simulink model "AltitudeControllerProject"  (R2026b)
settings: Solver=VariableStepAuto  StopTime=30
model workspace (MAT data in the model file):
  g = 9.81
  m = 1.5
undefined symbols (not defined in the file): Discrete, N, R, Time
libraries: slpidlib x1, ctrlSharedLib x1
settings Model: Creator=bosto  LastModifiedBy=bosto

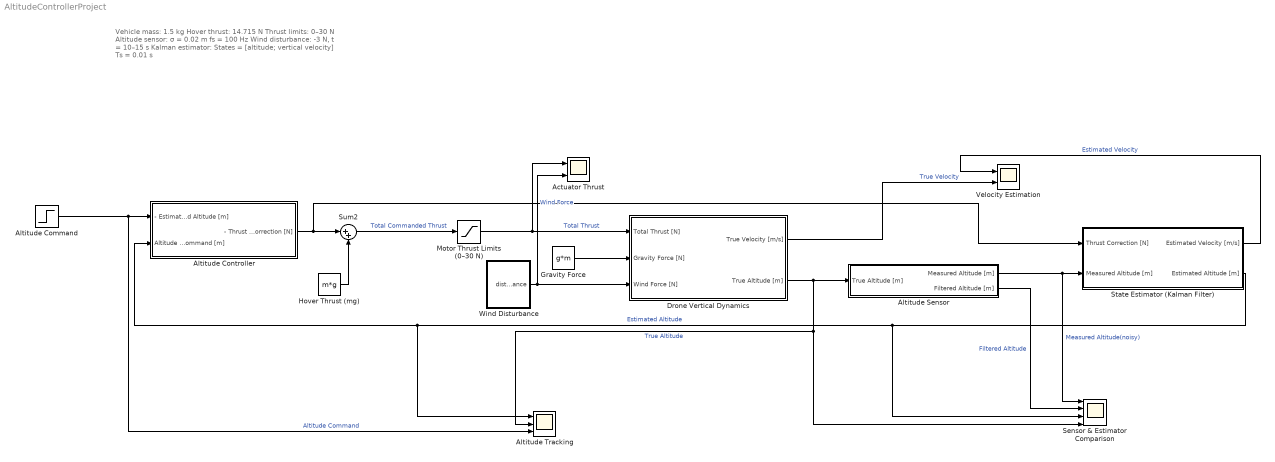
== system AltitudeControllerProject ==
  note: Vehicle mass: 1.5 kg
      | Hover thrust: 14.715 N
      | Thrust limits: 0–30 N
      |
      | Altitude sensor:
      | σ = 0.02 m
      | fs = 100 Hz
      |
      | Wind disturbance:
      | -3 N, t = 10–15 s
      |
      | Kalman estimator:
      | States = [altitude; vertical velocity]
      | Ts = 0.01 s
  Actuator Thrust : Scope  NumInputPorts=2
      settings: ActiveDisplayYMinimum=-7.1717687074829932  ActiveDisplayYMaximum=34.078231292517
  Altitude Command : Step  FinalValue=10  SampleTime=0
  Altitude Controller : Subsystem
  Altitude Sensor : Subsystem
  Altitude Tracking : Scope  NumInputPorts=3
      settings: ActiveDisplayYMinimum=-1.4089981765481037  ActiveDisplayYMaximum=12.477747899037325  DataLoggingVariableName=ScopeData3
  Drone Vertical Dynamics : Subsystem
  "Gravity Force " : Constant  Value=g*m
  Hover Thrust (mg) : Constant  Value=m*g
  Motor Thrust Limits (0–30 N) : Saturate  UpperLimit=30  LowerLimit=0
  Sensor & Estimator Comparison : Scope  NumInputPorts=4
      settings: ActiveDisplayYMinimum=9.9287970603381659  ActiveDisplayYMaximum=10.712908697624938
  State Estimator (Kalman Filter) : Subsystem
  Sum2 : Sum  Inputs=|++
  Velocity Estimation : Scope  NumInputPorts=2
      settings: ActiveDisplayYMinimum=-1.6989208652949748  ActiveDisplayYMaximum=10.973825126247741  DataLoggingVariableName=ScopeData4
  Wind Disturbance : Subsystem
  wires:
  Hover Thrust (mg)/1 -> Sum2/2
  "Gravity Force "/1 -> Drone Vertical Dynamics/2("Gravity Force [N] ")
  Motor Thrust Limits (0–30 N)/1 -> Actuator Thrust/1, Drone Vertical Dynamics/1(Total Thrust [N])  "Total Thrust"
  Sum2/1 -> Motor Thrust Limits (0–30 N)/1  "Total Commanded Thrust"
  Altitude Controller/1(- Thrust Correction [N]) -> Sum2/1, State Estimator (Kalman Filter)/1(Thrust Correction [N])
  Altitude Command/1 -> Altitude Tracking/3, Altitude Controller/1(- Estimated Altitude [m])  "Altitude Command"
  Altitude Sensor/2(Filtered Altitude [m]) -> Sensor & Estimator Comparison/2  "Filtered Altitude"
  Altitude Sensor/1(Measured Altitude [m]) -> Sensor & Estimator Comparison/1, State Estimator (Kalman Filter)/2(Measured Altitude [m])  "Measured Altitude(noisy)"
  State Estimator (Kalman Filter)/1(Estimated Velocity [m/s]) -> Velocity Estimation/1  "Estimated Velocity"
  State Estimator (Kalman Filter)/2(Estimated Altitude [m]) -> Sensor & Estimator Comparison/3, Altitude Tracking/1, Altitude Controller/2(Altitude Command [m])  "Estimated Altitude"
  Wind Disturbance/1(disturbance) -> Drone Vertical Dynamics/3(Wind Force [N]), Actuator Thrust/2  "Wind Force"
  Drone Vertical Dynamics/1(True Velocity [m/s]) -> Velocity Estimation/2  "True Velocity"
  Drone Vertical Dynamics/2(True Altitude [m]) -> Altitude Tracking/2, Sensor & Estimator Comparison/4, Altitude Sensor/1(True Altitude [m])  "True Altitude"

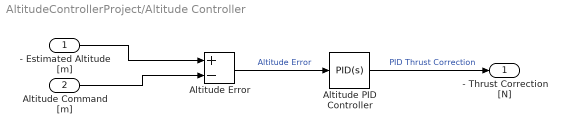
== system AltitudeControllerProject/Altitude Controller ==
  - Estimated Altitude [m] : Inport
  Altitude Command [m] : Inport  Port=2
  Altitude Error : Sum  Inputs=+-
  Altitude PID Controller : slpidlib/PID Controller  Controller=PID  Form=Parallel  TimeDomain=Continuous-time  UseExternalTs=off  SampleTime=-1  IntegratorMethod=Forward Euler  FilterMethod=Forward Euler  ControllerParametersSource=internal  P=34.1948073252816  I=4.38969736985132  UseKiTs=off  D=24.4181996821772  UseExternalDerivativeSource=off  N=10  UseFilter=on  TunerSelectOption=Transfer Function Based (PID Tuner App)  InitialConditionSource=internal  InitialConditionForIntegrator=0  InitialConditionForFilter=0  DifferentiatorICPrevScaledInput=0  ExternalReset=none  TrackingMode=off  Kt=1  LimitOutput=on  SatLimitsSource=internal  UpperSaturationLimit=15.285  LowerSaturationLimit=-14.715  LinearizeAsGain=on  AntiWindupMode=none  Kb=1  LimitIntegrator=off  UpperIntegratorSaturationLimit=inf  LowerIntegratorSaturationLimit=-inf  POutMin=[]  POutMax=[]  IOutMin=[]  IOutMax=[]  DOutMin=[]  DOutMax=[]  NOutMin=[]  NOutMax=[]  SumOutMin=[]  SumOutMax=[]  SaturationOutMin=[]  SaturationOutMax=[]  PParamMin=[]  PParamMax=[]  IParamMin=[]  IParamMax=[]  DParamMin=[]  DParamMax=[]  NParamMin=[]  NParamMax=[]  KbParamMin=[]  KbParamMax=[]  KtParamMin=[]  KtParamMax=[]  KbOutMin=[]  KbOutMax=[]  KtOutMin=[]  KtOutMax=[]  IntegratorOutMin=[]  IntegratorOutMax=[]  FilterOutMin=[]  FilterOutMax=[]  SumI1OutMin=[]  SumI1OutMax=[]  SumI2OutMin=[]  SumI2OutMax=[]  SumI3OutMin=[]  SumI3OutMax=[]  SumI4OutMin=[]  SumI4OutMax=[]  SumDOutMin=[]  SumDOutMax=[]  DifferentiatorOutMin=[]  DifferentiatorOutMax=[]  FilterDiffOutCoefMin=[]  FilterDiffOutCoefMax=[]  ReciprocalOutMin=[]  ReciprocalOutMax=[]  SumDenOutMin=[]  SumDenOutMax=[]  SumNumOutMin=[]  SumNumOutMax=[]  DivideOutMin=[]  DivideOutMax=[]  UdiffTsProdOutMin=[]  UdiffTsProdOutMax=[]  NTsProdOutMin=[]  NTsProdOutMax=[]  UintegralTsProdOutMin=[]  UintegralTsProdOutMax=[]  UngainTsProdOutMin=[]  UngainTsProdOutMax=[]  ClampingZeroOutDataTypeStr=Inherit: Inherit via back propagation  ClampingZeroOutMin=[]  ClampingZeroOutMax=[]  FilterDenConstantOutDataTypeStr=Inherit: Inherit via back propagation  FilterDenConstantOutMin=[]  FilterDenConstantOutMax=[]  PCopyOutDataTypeStr=Inherit: Inherit via back propagation  PCopyOutMin=[]  PCopyOutMax=[]  NCopyOutDataTypeStr=Inherit: Inherit via back propagation  NCopyOutMin=[]  NCopyOutMax=[]  IntegratorContinuousStateAttributes=''  IntegratorStateMustResolveToSignalObject=off  IntegratorRTWStateStorageClass=Auto  FilterContinuousStateAttributes=''  FilterStateMustResolveToSignalObject=off  FilterRTWStateStorageClass=Auto  ParallelPVariant=InternalParameters  IdealPVariant=Disabled  IVariant=InternalParameters  DVariant=InternalParameters  IntegratorVariant=Continuous  SatVariant=Enabled  AWVariant=Passthrough  PCopyVariant=Disabled  TRVariant=Disabled  FdbkBlocksVariant=Forward  IdealPFdbkVariant=Disabled  SatFdbkVariant=Disabled  DerivativeFilterVariant=ContFilter  NVariant=InternalParameters  NCopyVariant=Disabled  FilterICVariant=InternalICsFilter  IntegratorICVariant=InternalICs  ExternalResetVariant=Disabled  TRSumVariant=Passthrough  SumFdbkVariant=Disabled  SumVariant=Sum_PID  TsampFilterVariant=InternalTs  TsampNgainVariant=Passthrough  TsampIntegralVariant=Disabled_SignalSpec  ExternalSaturationOutDataTypeStr=Inherit: Same as second input  DerivativeSourceVariant=ErrorSignal  PreIntVariant=InternalPreInt
  - Thrust Correction [N] : Outport
  wires:
  - Estimated Altitude [m]/1 -> Altitude Error/1
  Altitude Error/1 -> Altitude PID Controller/1  "Altitude Error"
  Altitude Command [m]/1 -> Altitude Error/2
  Altitude PID Controller/1 -> - Thrust Correction [N]/1  "PID Thrust Correction"

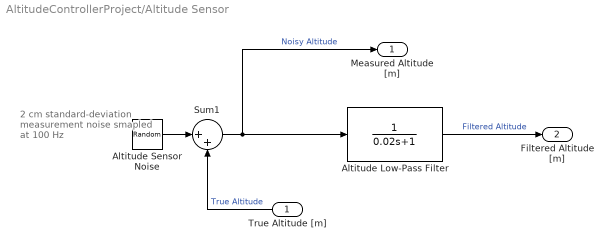
== system AltitudeControllerProject/Altitude Sensor ==
  note: 2 cm standard-deviation measurement noise smapled at 100 Hz
  True Altitude [m] : Inport
  Altitude Low-Pass Filter : TransferFcn  Denominator=[0.02 1]
  Altitude Sensor Noise : RandomNumber  Variance=0.0004  SampleTime=0.01
  Sum1 : Sum  Inputs=|++
  Measured Altitude [m] : Outport
  Filtered Altitude [m] : Outport  Port=2
  wires:
  True Altitude [m]/1 -> Sum1/2  "True Altitude"
  Altitude Sensor Noise/1 -> Sum1/1
  Altitude Low-Pass Filter/1 -> Filtered Altitude [m]/1  "Filtered Altitude"
  Sum1/1 -> Measured Altitude [m]/1, Altitude Low-Pass Filter/1  "Noisy Altitude"

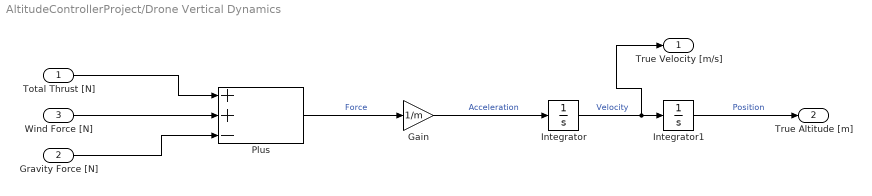
== system AltitudeControllerProject/Drone Vertical Dynamics ==
  Total Thrust [N] : Inport
  "Gravity Force [N] " : Inport  Port=2
  Wind Force [N] : Inport  Port=3
  Gain : Gain  Gain=1/m
  Integrator : Integrator
  Integrator1 : Integrator
  Plus : Sum  Inputs=++-
  True Velocity [m/s] : Outport
  True Altitude [m] : Outport  Port=2
  wires:
  Wind Force [N]/1 -> Plus/2
  Integrator1/1 -> True Altitude [m]/1  "Position"
  Gain/1 -> Integrator/1  "Acceleration"
  Plus/1 -> Gain/1  "Force"
  Integrator/1 -> True Velocity [m/s]/1, Integrator1/1  "Velocity"
  Total Thrust [N]/1 -> Plus/1
  "Gravity Force [N] "/1 -> Plus/3

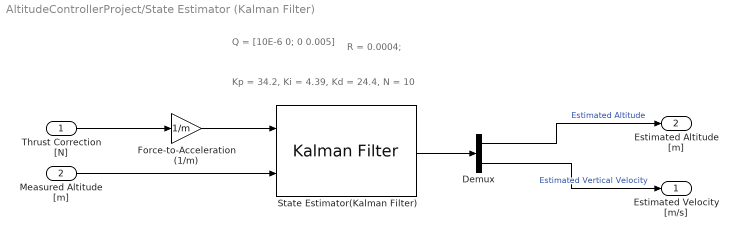
== system AltitudeControllerProject/State Estimator (Kalman Filter) ==
  note: Kp = 34.2, Ki = 4.39, Kd = 24.4, N = 10
  note: R = 0.0004;
  note: Q = [10E-6 0;
      | 0 0.005]
  Thrust Correction [N] : Inport
  Measured Altitude [m] : Inport  Port=2
  Demux : Demux  Outputs=2
  Force-to-Acceleration (1/m) : Gain  Gain=1/m
  State Estimator(Kalman Filter) : ctrlSharedLib/Kalman Filter  TimeDomain=Discrete-Time  UseCurrentEstimator=on  ModelSource=LTI State-Space Variable  ModelSourceVariable=droneEstimator  A=0.95  B=1  C=1  D=0  NumberOfStates=1  NumberOfInputs=1  NumberOfOutputs=1  Ts=-1  InitialEstimateSource=Dialog  X0=[0; 0]  P0=10  UseK=off  UseGH=off  G=1  TimeInvariantG=on  H=0  TimeInvariantH=on  NumberOfProcessNoiseInputs=1  Q=Q  TimeInvariantQ=on  R=R  TimeInvariantR=on  N=N  TimeInvariantN=on  AddInputPort=on  AddEnablePort=off  OutputEstimatedY=off  OutputP=off
  Estimated Velocity [m/s] : Outport
  Estimated Altitude [m] : Outport  Port=2
  wires:
  State Estimator(Kalman Filter)/1 -> Demux/1
  Measured Altitude [m]/1 -> State Estimator(Kalman Filter)/2
  Demux/2 -> Estimated Velocity [m/s]/1  "Estimated Vertical Velocity"
  Demux/1 -> Estimated Altitude [m]/1  "Estimated Altitude"
  Force-to-Acceleration (1/m)/1 -> State Estimator(Kalman Filter)/1
  Thrust Correction [N]/1 -> Force-to-Acceleration (1/m)/1

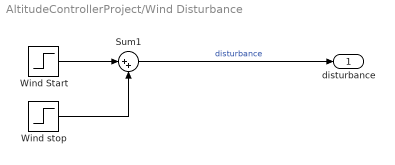
== system AltitudeControllerProject/Wind Disturbance ==
  Sum1 : Sum  Inputs=|++
  Wind Start : Step  Time=10  FinalValue=-3  SampleTime=0
  Wind stop : Step  Time=15  FinalValue=3  SampleTime=0
  disturbance : Outport
  wires:
  Wind Start/1 -> Sum1/1
  Sum1/1 -> disturbance/1  "disturbance"
  Wind stop/1 -> Sum1/2
